simulink model "sg"  (R2021b)
settings: Solver=ode4  StartTime=0.0  StopTime=10  FixedStep=Ts  RelTol=1e-3  EnableMultiTasking=on
model workspace (MAT data in the model file):
  AU1 = 0.174532925199
  AU2 = 0
  AU3 = 0
  AW = 0
  FU1 = 0.1
  FU2 = 0
  FU3 = 0
  FW = 0
  GainU1 = 1
  GainU2 = 1
  GainU3 = 1
  GainW = 1
  KD1 = 0
  KD2 = 0
  KD3 = 0
  KI1 = 0
  KI2 = 0
  KI3 = 0
  KP1 = 1
  KP2 = 1
  KP3 = 1
  N1 = 100
  N2 = 100
  N3 = 100
  SatU1 = 0.174532920122
  SatU2 = 0.174532920122
  SatU3 = 0.174532920122
  SatW = 0.300000011921
  controlMode = 0
  qref = [0.698131680489; -0.523598790169; -1.57079637051]
libraries: slpidlib x3, slrealtimeutilitieslib x2, slrealtimeiplib x2
settings Model: Creator=ronnyl10  LastModifiedBy=Mechatronics_lab
settings SolverCC: ConcurrentTasks=on  AlgebraicLoopSolver=TrustRegion  PositivePriorityOrder=on  InsertRTBMode=Never (minimum delay)
settings DataIOCC: ExternalInput=ds  LoadExternalInput=on  SaveFormat=Array  SaveState=on  SignalLoggingName=logsOut
settings OptimizationCC: BlockReduction=off  BooleanDataType=off  OptimizeBlockIOStorage=off  BufferReuse=off  GlobalBufferReuse=off  ExpressionFolding=off  LocalBlockOutputs=off  InitFltsAndDblsToZero=on  OptimizeDataStoreBuffers=off  BusAssignmentInplaceUpdate=off
settings DebuggingCC: SaveWithParameterizedLinksMsg=none  UnderspecifiedInitializationDetection=Classic  MergeDetectMultiDrivingBlocksExec=none  CheckExecutionContextPreStartOutputMsg=on  SignalResolutionControl=TryResolveAllWithWarning  TasksWithSamePriorityMsg=none  SFUnexpectedBacktrackingDiag=warning  SFNoUnconditionalDefaultTransitionDiag=warning  SFExecutionAtInitializationDiag=none  SFMachineParentedDataDiag=warning  ArithmeticOperatorsInVariantConditions=warning
settings HardwareCC: ProdBitPerLong=64  ProdLongLongMode=on  ProdHWDeviceType=Intel->x86-64 (Linux 64)
settings ModelReferenceCC: PropagateSignalLabelsOutOfModel=off
settings SFSimCC: SimUseLocalCustomCode=off  SimTargetLang=C++
settings RTWCC: Description=Simulink Real-Time  SystemTargetFile=slrealtime.tlc  TemplateMakefile=slrealtime_default_tmf  RTWVerbose=off  RTWUseLocalCustomCode=off  Toolchain=Simulink Real-Time Toolchain  BuildConfiguration=Faster Runs  CodeExecutionProfiling=on  TargetLang=C++
settings CodeAppCC: StateflowObjectComments=on
settings SimulinkRealTimeTargetCC: MATLABClassNameForMDSCustomization=Simulink.SoftwareTarget.GRTCustomization  UseGCCFastMath=on
settings ConfigComp: CovMetricSettings=dw  CovSaveCumulativeToWorkspaceVar=on  CovSaveSingleToWorkspaceVar=on  CovExternalEMLEnable=off  CovSFcnEnable=off

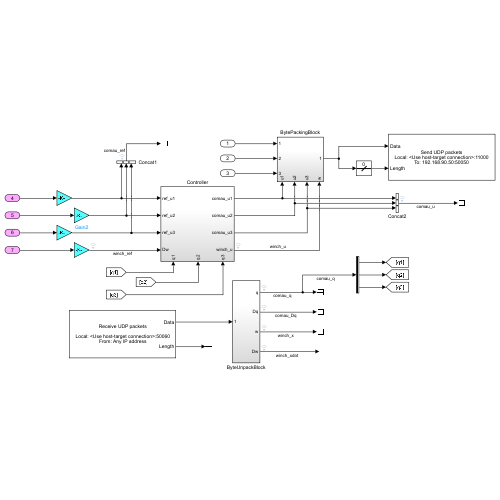
[thumbnail: Simulink's stored preview of the top-level diagram]
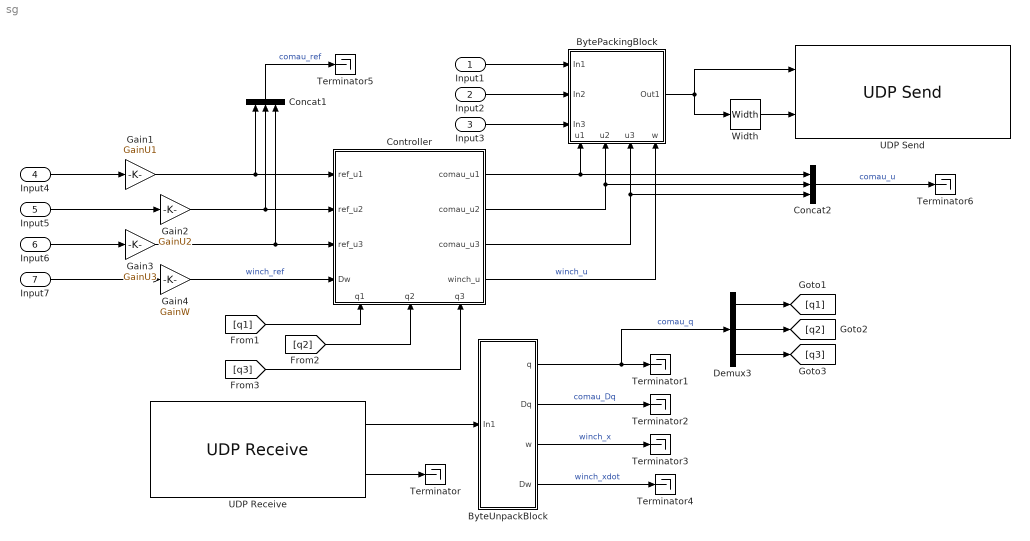
== system sg ==
  Input1 : Inport  OutDataTypeStr=uint32
  Input2 : Inport  Port=2  OutDataTypeStr=single
  Input3 : Inport  Port=3  OutDataTypeStr=single
  Input4 : Inport  Port=4  OutDataTypeStr=single  LockScale=on
  Input5 : Inport  Port=5  OutDataTypeStr=single  LockScale=on
  Input6 : Inport  Port=6  OutDataTypeStr=single  LockScale=on
  Input7 : Inport  Port=7  OutDataTypeStr=single
  BytePackingBlock : Subsystem
      settings: PortSchema="{\"entries\":[{\"content\":{\"sides\":[{\"content\":{\"connectorIds\":[\"In1\",\"In2\",\"In3\"]},\"type\":\"ConnectorPlacement.EquallySpacedRectSide\",\"uuid\":\"2ce4a3a0-ffcc-43d7-9a0a-8eda699e79f7\"},{\"content\":{\"connectorIds\":[\"Out1\"],\"side\":\"RIGHT\"},\"type\":\"ConnectorPlacement.EquallySpacedRectSide\",\"uuid\":\"6b0835cb-1c02-4104-b44f-3bd25ad1f1a4\"},{\"content\":{\"connectorIds\":[],\"side\":\"TOP\"},\"type\":\"ConnectorPlacement.EquallySpacedRectSide\",\"uuid\":\"5708f016-a603-4602-bfb0-c60eac1ca3fe\"},{\"content\":{\"connectorIds\":[\"In4\",\"In5\",\"In6\",\"In7\"],\"side\":\"BOTTOM\"},\"type\":\"ConnectorPlacement.EquallySpacedRectSide\",\"uuid\":\"ec76ed57-869b-40d0-9db7-9ec796597bae\"}]},\"type\":\"ConnectorPlacement.EquallySpacedConnector\",\"uuid\":\"dfe3046e-e9d4-4a64-bd13-28ebfaf09d3c\"}],\"packageUris\":[\"http://schema.mathworks.com/mf0/Connector/R2020b\"],\"version\":\"1.0\"}"
  ByteUnpackBlock : Subsystem
  Concat1 : Concatenate  NumInputs=3  ConcatenateDimension=2
  Concat2 : Concatenate  NumInputs=3  ConcatenateDimension=2
  Controller : Subsystem
      settings: PortSchema="{\"entries\":[{\"content\":{\"sides\":[{\"content\":{\"connectorIds\":[\"In1\",\"In2\",\"In3\",\"In4\"]},\"type\":\"ConnectorPlacement.EquallySpacedRectSide\",\"uuid\":\"8cd68c6a-417b-4593-9fd2-f26242799ae2\"},{\"content\":{\"connectorIds\":[\"Out1\",\"Out2\",\"Out3\",\"Out4\"],\"side\":\"RIGHT\"},\"type\":\"ConnectorPlacement.EquallySpacedRectSide\",\"uuid\":\"847d4d9d-1a2d-44bd-a0b5-d0f29db0c6e7\"},{\"content\":{\"connectorIds\":[],\"side\":\"TOP\"},\"type\":\"ConnectorPlacement.EquallySpacedRectSide\",\"uuid\":\"bbe996aa-4357-46c2-b640-27c97a1f9741\"},{\"content\":{\"connectorIds\":[\"In5\",\"In6\",\"In7\"],\"side\":\"BOTTOM\"},\"type\":\"ConnectorPlacement.EquallySpacedRectSide\",\"uuid\":\"3733f1bb-3723-42d5-ab99-3fe4b1c5b9a3\"}]},\"type\":\"ConnectorPlacement.EquallySpacedConnector\",\"uuid\":\"cdb9b215-90f3-4ef7-bdcb-b6cb1e13a832\"}],\"packageUris\":[\"http://schema.mathworks.com/mf0/Connector/R2020b\"],\"version\":\"1.0\"}"
  Demux3 : Demux  Outputs=3
  Gain1 : Gain  Gain=GainU1  OutDataTypeStr=single
  Gain2 : Gain  Gain=GainU2  OutDataTypeStr=single
  Gain3 : Gain  Gain=GainU3  OutDataTypeStr=single
  Gain4 : Gain  Gain=GainW  OutDataTypeStr=single
  Terminator{,1..6} (7 alike) : Terminator
  UDP Receive : slrealtimeiplib/UDP Receive  useHostTargetConn=on  ipAddress=192.168.90.60  localPort=50060  rcvWidth=304  rcvFmAny=on  fmAddress=192.168.90.50  sampleTime=Ts
      settings: SourceProductBaseCode=XP
  UDP Send : slrealtimeiplib/UDP Send  useHostTargetConn=on  toAddress=192.168.90.50  toPort=50050  sampleTime=Ts  localPort=11000
      settings: SourceProductBaseCode=XP
  Width : Width
  wires:
  Width/1 -> UDP Send/2
  UDP Receive/2 -> Terminator/1
  Concat2/1 -> Terminator6/1  "comau_u"
  BytePackingBlock/1(Out1) -> Width/1, UDP Send/1
  Input1/1 -> BytePackingBlock/1(In1)
  Input3/1 -> BytePackingBlock/3(In3)
  Input2/1 -> BytePackingBlock/2(In2)
  UDP Receive/1 -> ByteUnpackBlock/1(In1)
  Input4/1 -> Gain1/1
  Input5/1 -> Gain2/1
  Input6/1 -> Gain3/1
  ByteUnpackBlock/3(w) -> Terminator3/1  "winch_x"
  ByteUnpackBlock/4(Dw) -> Terminator4/1  "winch_xdot"
  Controller/3(comau_u3) -> Concat2/3, BytePackingBlock/6(u3)
  Controller/2(comau_u2) -> Concat2/2, BytePackingBlock/5(u2)
  Controller/1(comau_u1) -> BytePackingBlock/4(u1), Concat2/1
  Concat1/1 -> Terminator5/1  "comau_ref"
  Controller/4(winch_u) -> BytePackingBlock/7(w)  "winch_u"
  ByteUnpackBlock/2(Dq) -> Terminator2/1  "comau_Dq"
  Input7/1 -> Gain4/1
  Gain4/1 -> Controller/4(Dw)  "winch_ref"
  Gain1/1 -> Concat1/1, Controller/1(ref_u1)
  Gain2/1 -> Controller/2(ref_u2), Concat1/2
  Gain3/1 -> Concat1/3, Controller/3(ref_u3)
  ByteUnpackBlock/1(q) -> Demux3/1, Terminator1/1  "comau_q"
  Demux3/1 -> [q1]
  Demux3/2 -> [q2]
  Demux3/3 -> [q3]
  [q2] -> Controller/6(q2)
  [q3] -> Controller/7(q3)
  [q1] -> Controller/5(q1)

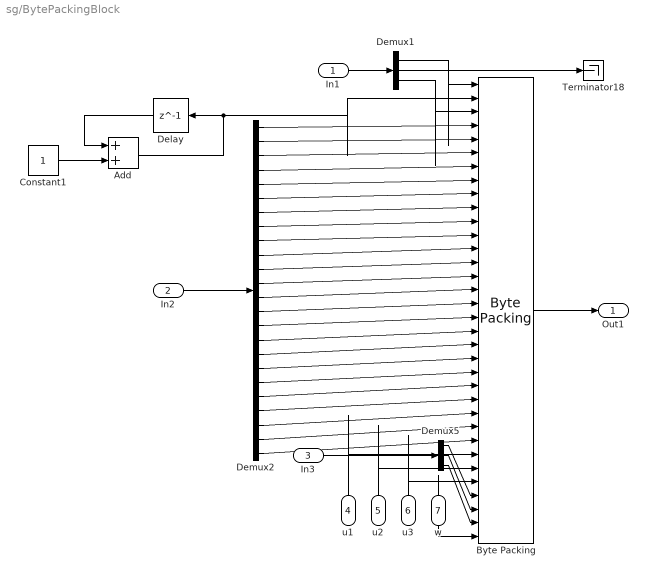
== system sg/BytePackingBlock ==
  In1 : Inport
  In2 : Inport  Port=2
  In3 : Inport  Port=3
  u1 : Inport  Port=4
  u2 : Inport  Port=5
  u3 : Inport  Port=6
  w : Inport  Port=7
  Add : Sum
  Byte Packing : slrealtimeutilitieslib/Byte Packing  MaskPackedDataType=uint8  MaskUnpackedDataTypes={'uint32', 'uint32', 'uint32', 'single', 'single', 'single', 'single', 'single', 'single', 'single', 'single', 'single', 'single', 'single', 'single', 'single', 'single', 'single', 'single', 'single', 'single', 'single', 'single', 'single', 'single', 'single', 'single', 'single', 'single', 'single', 'single', 'single', 'single', 'single'}  MaskAlignment=1
  Constant1 : Constant  OutDataTypeStr=uint32
  Delay : Delay  DelayLength=1
  Demux1 : Demux  Outputs=3
  Demux2 : Demux  Outputs=24
  Demux5 : Demux  Outputs=3
  Terminator18 : Terminator
  Out1 : Outport
  wires:
  Demux2/19 -> Byte Packing/22
  Demux2/21 -> Byte Packing/24
  u3/1 -> Byte Packing/30
  Demux2/2 -> Byte Packing/5
  u2/1 -> Byte Packing/29
  Demux5/1 -> Byte Packing/31
  Demux5/2 -> Byte Packing/32
  Demux1/3 -> Byte Packing/3
  In2/1 -> Demux2/1
  Demux2/22 -> Byte Packing/25
  Demux2/1 -> Byte Packing/4
  Demux2/15 -> Byte Packing/18
  Demux2/18 -> Byte Packing/21
  Delay/1 -> Add/1
  Demux2/24 -> Byte Packing/27
  Demux1/2 -> Terminator18/1
  In1/1 -> Demux1/1
  Demux2/5 -> Byte Packing/8
  Add/1 -> Byte Packing/2, Delay/1
  Constant1/1 -> Add/2
  Demux2/6 -> Byte Packing/9
  Demux2/9 -> Byte Packing/12
  Demux2/10 -> Byte Packing/13
  Demux2/20 -> Byte Packing/23
  Demux2/8 -> Byte Packing/11
  Demux2/12 -> Byte Packing/15
  Demux2/23 -> Byte Packing/26
  Demux2/16 -> Byte Packing/19
  Demux1/1 -> Byte Packing/1
  Demux5/3 -> Byte Packing/33
  Demux2/3 -> Byte Packing/6
  Demux2/11 -> Byte Packing/14
  Demux2/7 -> Byte Packing/10
  Demux2/4 -> Byte Packing/7
  Demux2/13 -> Byte Packing/16
  Demux2/17 -> Byte Packing/20
  Demux2/14 -> Byte Packing/17
  u1/1 -> Byte Packing/28
  In3/1 -> Demux5/1
  Byte Packing/1 -> Out1/1
  w/1 -> Byte Packing/34

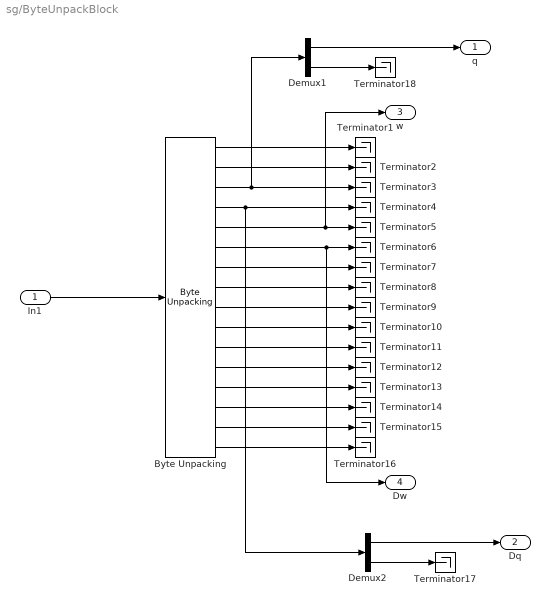
== system sg/ByteUnpackBlock ==
  In1 : Inport
  Byte Unpacking : slrealtimeutilitieslib/Byte Unpacking  MaskUnpackedDataTypes={'uint32', 'single', 'single', 'single', 'single', 'single', 'single', 'single', 'single', 'single', 'single', 'single', 'single', 'single', 'single', 'single'}  MaskUnpackedDataSizes={[1], [1], [6], [6], [1], [1], [6], [6], [6], [6], [6], [6], [6], [6], [6], [6]}  MaskAlignment=1
      settings: SourceProductBaseCode=XP
  Demux1 : Demux  Outputs=2
  Demux2 : Demux  Outputs=2
  Terminator{1..18} (18 alike) : Terminator
  q : Outport
  Dq : Outport  Port=2
  w : Outport  Port=3
  Dw : Outport  Port=4
  wires:
  Byte Unpacking/13 -> Terminator13/1
  Byte Unpacking/8 -> Terminator8/1
  Byte Unpacking/1 -> Terminator1/1
  Byte Unpacking/7 -> Terminator7/1
  Byte Unpacking/16 -> Terminator16/1
  Byte Unpacking/6 -> Terminator6/1, Dw/1
  Byte Unpacking/11 -> Terminator11/1
  Byte Unpacking/10 -> Terminator10/1
  Byte Unpacking/15 -> Terminator15/1
  Byte Unpacking/2 -> Terminator2/1
  Byte Unpacking/14 -> Terminator14/1
  Byte Unpacking/5 -> w/1, Terminator5/1
  Byte Unpacking/9 -> Terminator9/1
  Byte Unpacking/12 -> Terminator12/1
  In1/1 -> Byte Unpacking/1
  Demux1/1 -> q/1
  Byte Unpacking/3 -> Demux1/1, Terminator3/1
  Demux2/1 -> Dq/1
  Byte Unpacking/4 -> Demux2/1, Terminator4/1
  Demux1/2 -> Terminator18/1
  Demux2/2 -> Terminator17/1

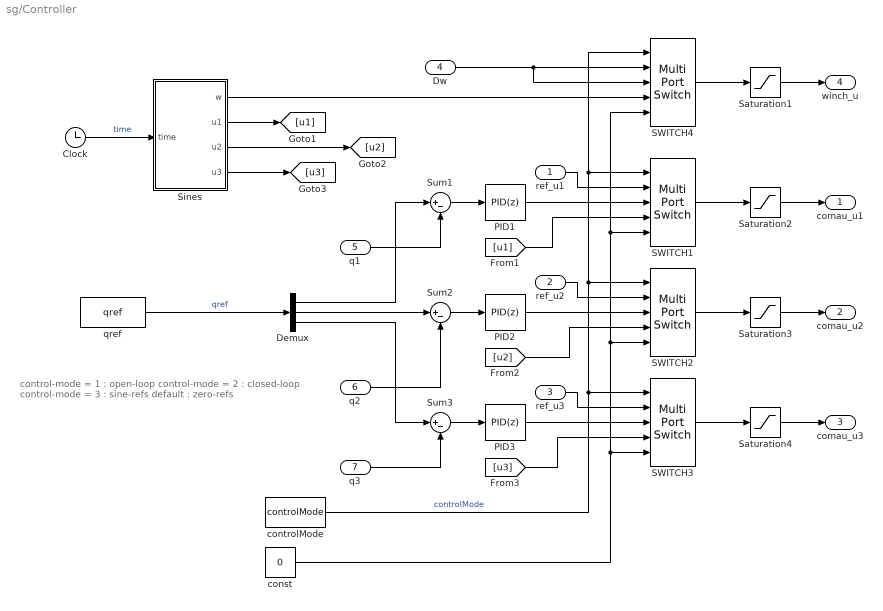
== system sg/Controller ==
  note: control-mode = 1 : open-loop
      | control-mode = 2 : closed-loop
      | control-mode = 3 : sine-refs
      | default : zero-refs
  ref_u1 : Inport
  ref_u2 : Inport  Port=2
  ref_u3 : Inport  Port=3
  Dw : Inport  Port=4
  q1 : Inport  Port=5
  q2 : Inport  Port=6
  q3 : Inport  Port=7
  Clock : Clock
  Demux : Demux  Outputs=3
  PID1 : slpidlib/PID Controller  Controller=PID  Form=Parallel  TimeDomain=Discrete-time  UseExternalTs=off  SampleTime=-1  IntegratorMethod=Forward Euler  FilterMethod=Forward Euler  ControllerParametersSource=internal  P=KP1  I=KI1  D=KD1  UseFilter=on  N=N1  TunerSelectOption=Transfer Function Based (PID Tuner App)  InitialConditionSource=internal  InitialConditionForIntegrator=0  InitialConditionForFilter=0  DifferentiatorICPrevScaledInput=0  ExternalReset=none  TrackingMode=off  Kt=1  LimitOutput=off  SatLimitsSource=internal  UpperSaturationLimit=inf  LowerSaturationLimit=-inf  LinearizeAsGain=on  AntiWindupMode=none  Kb=1  POutMin=[]  POutMax=[]  IOutMin=[]  IOutMax=[]  DOutMin=[]  DOutMax=[]  NOutMin=[]  NOutMax=[]  SumOutMin=[]  SumOutMax=[]  SaturationOutMin=[]  SaturationOutMax=[]  PParamMin=[]  PParamMax=[]  IParamMin=[]  IParamMax=[]  DParamMin=[]  DParamMax=[]  NParamMin=[]  NParamMax=[]  KbParamMin=[]  KbParamMax=[]  KtParamMin=[]  KtParamMax=[]  KbOutMin=[]  KbOutMax=[]  KtOutMin=[]  KtOutMax=[]  IntegratorOutMin=[]  IntegratorOutMax=[]  FilterOutMin=[]  FilterOutMax=[]  SumI1OutMin=[]  SumI1OutMax=[]  SumI2OutMin=[]  SumI2OutMax=[]  SumI3OutMin=[]  SumI3OutMax=[]  SumI4OutMin=[]  SumI4OutMax=[]  SumDOutMin=[]  SumDOutMax=[]  DifferentiatorOutMin=[]  DifferentiatorOutMax=[]  FilterDiffOutCoefMin=[]  FilterDiffOutCoefMax=[]  ReciprocalOutMin=[]  ReciprocalOutMax=[]  SumDenOutMin=[]  SumDenOutMax=[]  SumNumOutMin=[]  SumNumOutMax=[]  DivideOutMin=[]  DivideOutMax=[]  UdiffTsProdOutMin=[]  UdiffTsProdOutMax=[]  NTsProdOutMin=[]  NTsProdOutMax=[]  UintegralTsProdOutMin=[]  UintegralTsProdOutMax=[]  UngainTsProdOutMin=[]  UngainTsProdOutMax=[]  FilterDenConstantOutDataTypeStr=Inherit: Inherit via back propagation  FilterDenConstantOutMin=[]  FilterDenConstantOutMax=[]  PCopyOutDataTypeStr=Inherit: Inherit via back propagation  PCopyOutMin=[]  PCopyOutMax=[]  NCopyOutDataTypeStr=Inherit: Inherit via back propagation  NCopyOutMin=[]  NCopyOutMax=[]  IntegratorContinuousStateAttributes=''  IntegratorStateMustResolveToSignalObject=off  IntegratorRTWStateStorageClass=Auto  FilterContinuousStateAttributes=''  FilterStateMustResolveToSignalObject=off  FilterRTWStateStorageClass=Auto  ParallelPVariant=InternalParameters  IdealPVariant=Disabled  IVariant=InternalParameters  DVariant=InternalParameters  IntegratorVariant=Discrete  SatVariant=Disabled  AWVariant=Passthrough  PCopyVariant=Disabled  TRVariant=Disabled  FdbkBlocksVariant=Forward  IdealPFdbkVariant=Disabled  SatFdbkVariant=Disabled  DerivativeFilterVariant=ForwardEulerFilter  NVariant=InternalParameters  NCopyVariant=Disabled  FilterICVariant=InternalICsFilter  IntegratorICVariant=InternalICs  ExternalResetVariant=Disabled  TRSumVariant=Passthrough  SumFdbkVariant=Disabled  SumVariant=Sum_PID  TsampFilterVariant=InternalTs  TsampNgainVariant=Passthrough  TsampIntegralVariant=Passthrough  ExternalSaturationOutDataTypeStr=Inherit: Same as second input
  PID2 : slpidlib/PID Controller  Controller=PID  Form=Parallel  TimeDomain=Discrete-time  UseExternalTs=off  SampleTime=-1  IntegratorMethod=Forward Euler  FilterMethod=Forward Euler  ControllerParametersSource=internal  P=KP2  I=KI2  D=KD2  UseFilter=on  N=N2  TunerSelectOption=Transfer Function Based (PID Tuner App)  InitialConditionSource=internal  InitialConditionForIntegrator=0  InitialConditionForFilter=0  DifferentiatorICPrevScaledInput=0  ExternalReset=none  TrackingMode=off  Kt=1  LimitOutput=off  SatLimitsSource=internal  UpperSaturationLimit=inf  LowerSaturationLimit=-inf  LinearizeAsGain=on  AntiWindupMode=none  Kb=1  POutMin=[]  POutMax=[]  IOutMin=[]  IOutMax=[]  DOutMin=[]  DOutMax=[]  NOutMin=[]  NOutMax=[]  SumOutMin=[]  SumOutMax=[]  SaturationOutMin=[]  SaturationOutMax=[]  PParamMin=[]  PParamMax=[]  IParamMin=[]  IParamMax=[]  DParamMin=[]  DParamMax=[]  NParamMin=[]  NParamMax=[]  KbParamMin=[]  KbParamMax=[]  KtParamMin=[]  KtParamMax=[]  KbOutMin=[]  KbOutMax=[]  KtOutMin=[]  KtOutMax=[]  IntegratorOutMin=[]  IntegratorOutMax=[]  FilterOutMin=[]  FilterOutMax=[]  SumI1OutMin=[]  SumI1OutMax=[]  SumI2OutMin=[]  SumI2OutMax=[]  SumI3OutMin=[]  SumI3OutMax=[]  SumI4OutMin=[]  SumI4OutMax=[]  SumDOutMin=[]  SumDOutMax=[]  DifferentiatorOutMin=[]  DifferentiatorOutMax=[]  FilterDiffOutCoefMin=[]  FilterDiffOutCoefMax=[]  ReciprocalOutMin=[]  ReciprocalOutMax=[]  SumDenOutMin=[]  SumDenOutMax=[]  SumNumOutMin=[]  SumNumOutMax=[]  DivideOutMin=[]  DivideOutMax=[]  UdiffTsProdOutMin=[]  UdiffTsProdOutMax=[]  NTsProdOutMin=[]  NTsProdOutMax=[]  UintegralTsProdOutMin=[]  UintegralTsProdOutMax=[]  UngainTsProdOutMin=[]  UngainTsProdOutMax=[]  FilterDenConstantOutDataTypeStr=Inherit: Inherit via back propagation  FilterDenConstantOutMin=[]  FilterDenConstantOutMax=[]  PCopyOutDataTypeStr=Inherit: Inherit via back propagation  PCopyOutMin=[]  PCopyOutMax=[]  NCopyOutDataTypeStr=Inherit: Inherit via back propagation  NCopyOutMin=[]  NCopyOutMax=[]  IntegratorContinuousStateAttributes=''  IntegratorStateMustResolveToSignalObject=off  IntegratorRTWStateStorageClass=Auto  FilterContinuousStateAttributes=''  FilterStateMustResolveToSignalObject=off  FilterRTWStateStorageClass=Auto  ParallelPVariant=InternalParameters  IdealPVariant=Disabled  IVariant=InternalParameters  DVariant=InternalParameters  IntegratorVariant=Discrete  SatVariant=Disabled  AWVariant=Passthrough  PCopyVariant=Disabled  TRVariant=Disabled  FdbkBlocksVariant=Forward  IdealPFdbkVariant=Disabled  SatFdbkVariant=Disabled  DerivativeFilterVariant=ForwardEulerFilter  NVariant=InternalParameters  NCopyVariant=Disabled  FilterICVariant=InternalICsFilter  IntegratorICVariant=InternalICs  ExternalResetVariant=Disabled  TRSumVariant=Passthrough  SumFdbkVariant=Disabled  SumVariant=Sum_PID  TsampFilterVariant=InternalTs  TsampNgainVariant=Passthrough  TsampIntegralVariant=Passthrough  ExternalSaturationOutDataTypeStr=Inherit: Same as second input
  PID3 : slpidlib/PID Controller  Controller=PID  Form=Parallel  TimeDomain=Discrete-time  UseExternalTs=off  SampleTime=-1  IntegratorMethod=Forward Euler  FilterMethod=Forward Euler  ControllerParametersSource=internal  P=KP3  I=KI3  D=KD3  UseFilter=on  N=N3  TunerSelectOption=Transfer Function Based (PID Tuner App)  InitialConditionSource=internal  InitialConditionForIntegrator=0  InitialConditionForFilter=0  DifferentiatorICPrevScaledInput=0  ExternalReset=none  TrackingMode=off  Kt=1  LimitOutput=off  SatLimitsSource=internal  UpperSaturationLimit=inf  LowerSaturationLimit=-inf  LinearizeAsGain=on  AntiWindupMode=none  Kb=1  POutMin=[]  POutMax=[]  IOutMin=[]  IOutMax=[]  DOutMin=[]  DOutMax=[]  NOutMin=[]  NOutMax=[]  SumOutMin=[]  SumOutMax=[]  SaturationOutMin=[]  SaturationOutMax=[]  PParamMin=[]  PParamMax=[]  IParamMin=[]  IParamMax=[]  DParamMin=[]  DParamMax=[]  NParamMin=[]  NParamMax=[]  KbParamMin=[]  KbParamMax=[]  KtParamMin=[]  KtParamMax=[]  KbOutMin=[]  KbOutMax=[]  KtOutMin=[]  KtOutMax=[]  IntegratorOutMin=[]  IntegratorOutMax=[]  FilterOutMin=[]  FilterOutMax=[]  SumI1OutMin=[]  SumI1OutMax=[]  SumI2OutMin=[]  SumI2OutMax=[]  SumI3OutMin=[]  SumI3OutMax=[]  SumI4OutMin=[]  SumI4OutMax=[]  SumDOutMin=[]  SumDOutMax=[]  DifferentiatorOutMin=[]  DifferentiatorOutMax=[]  FilterDiffOutCoefMin=[]  FilterDiffOutCoefMax=[]  ReciprocalOutMin=[]  ReciprocalOutMax=[]  SumDenOutMin=[]  SumDenOutMax=[]  SumNumOutMin=[]  SumNumOutMax=[]  DivideOutMin=[]  DivideOutMax=[]  UdiffTsProdOutMin=[]  UdiffTsProdOutMax=[]  NTsProdOutMin=[]  NTsProdOutMax=[]  UintegralTsProdOutMin=[]  UintegralTsProdOutMax=[]  UngainTsProdOutMin=[]  UngainTsProdOutMax=[]  FilterDenConstantOutDataTypeStr=Inherit: Inherit via back propagation  FilterDenConstantOutMin=[]  FilterDenConstantOutMax=[]  PCopyOutDataTypeStr=Inherit: Inherit via back propagation  PCopyOutMin=[]  PCopyOutMax=[]  NCopyOutDataTypeStr=Inherit: Inherit via back propagation  NCopyOutMin=[]  NCopyOutMax=[]  IntegratorContinuousStateAttributes=''  IntegratorStateMustResolveToSignalObject=off  IntegratorRTWStateStorageClass=Auto  FilterContinuousStateAttributes=''  FilterStateMustResolveToSignalObject=off  FilterRTWStateStorageClass=Auto  ParallelPVariant=InternalParameters  IdealPVariant=Disabled  IVariant=InternalParameters  DVariant=InternalParameters  IntegratorVariant=Discrete  SatVariant=Disabled  AWVariant=Passthrough  PCopyVariant=Disabled  TRVariant=Disabled  FdbkBlocksVariant=Forward  IdealPFdbkVariant=Disabled  SatFdbkVariant=Disabled  DerivativeFilterVariant=ForwardEulerFilter  NVariant=InternalParameters  NCopyVariant=Disabled  FilterICVariant=InternalICsFilter  IntegratorICVariant=InternalICs  ExternalResetVariant=Disabled  TRSumVariant=Passthrough  SumFdbkVariant=Disabled  SumVariant=Sum_PID  TsampFilterVariant=InternalTs  TsampNgainVariant=Passthrough  TsampIntegralVariant=Passthrough  ExternalSaturationOutDataTypeStr=Inherit: Same as second input
  SWITCH1 : MultiPortSwitch  DataPortForDefault=Additional data port
  SWITCH2 : MultiPortSwitch  DataPortForDefault=Additional data port
  SWITCH3 : MultiPortSwitch  DataPortForDefault=Additional data port
  SWITCH4 : MultiPortSwitch  DataPortIndices={1,3}  DataPortForDefault=Additional data port
  Saturation1 : Saturate  UpperLimit=SatW  LowerLimit=-SatW
  Saturation2 : Saturate  UpperLimit=SatU1  LowerLimit=-SatU1
  Saturation3 : Saturate  UpperLimit=SatU2  LowerLimit=-SatU2
  Saturation4 : Saturate  UpperLimit=SatU3  LowerLimit=-SatU3
  Sines : Subsystem
  Sum1 : Sum  Inputs=|+-
  Sum2 : Sum  Inputs=|+-
  Sum3 : Sum  Inputs=|+-
  const : Constant  Value=0  OutDataTypeStr=single
  controlMode : Constant  Value=controlMode  OutDataTypeStr=double
  qref : Constant  Value=qref
  comau_u1 : Outport
  comau_u2 : Outport  Port=2
  comau_u3 : Outport  Port=3
  winch_u : Outport  Port=4
  wires:
  Saturation1/1 -> winch_u/1
  Saturation2/1 -> comau_u1/1
  Saturation3/1 -> comau_u2/1
  Saturation4/1 -> comau_u3/1
  q2/1 -> Sum2/2
  q3/1 -> Sum3/2
  Demux/1 -> Sum1/1
  q1/1 -> Sum1/2
  Sum1/1 -> PID1/1
  Sum2/1 -> PID2/1
  PID3/1 -> SWITCH3/3
  Demux/3 -> Sum3/1
  Sum3/1 -> PID3/1
  [u3] -> SWITCH3/4
  PID2/1 -> SWITCH2/3
  [u2] -> SWITCH2/4
  PID1/1 -> SWITCH1/3
  [u1] -> SWITCH1/4
  const/1 -> SWITCH4/5, SWITCH1/5, SWITCH2/5, SWITCH3/5
  SWITCH4/1 -> Saturation1/1
  SWITCH1/1 -> Saturation2/1
  SWITCH2/1 -> Saturation3/1
  SWITCH3/1 -> Saturation4/1
  Dw/1 -> SWITCH4/3, SWITCH4/2
  controlMode/1 -> SWITCH3/1, SWITCH2/1, SWITCH4/1, SWITCH1/1  "controlMode"
  ref_u1/1 -> SWITCH1/2
  qref/1 -> Demux/1  "qref"
  ref_u2/1 -> SWITCH2/2
  ref_u3/1 -> SWITCH3/2
  Demux/2 -> Sum2/1
  Clock/1 -> Sines/1(time)  "time"
  Sines/2(u1) -> [u1]
  Sines/1(w) -> SWITCH4/4
  Sines/3(u2) -> [u2]
  Sines/4(u3) -> [u3]

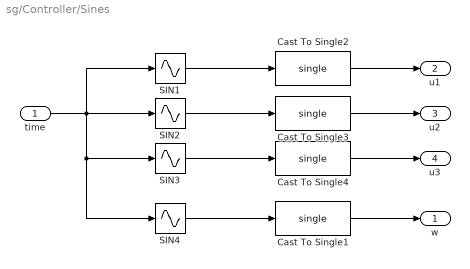
== system sg/Controller/Sines ==
  time : Inport
  Cast To Single{1..4} (4 alike) : DataTypeConversion  OutDataTypeStr=single
  SIN1 : Sin  TimeSource=Use external signal  Amplitude=AU1  Frequency=FU1*2*pi  SampleTime=0
  SIN2 : Sin  TimeSource=Use external signal  Amplitude=AU2  Frequency=FU2*2*pi  SampleTime=0
  SIN3 : Sin  TimeSource=Use external signal  Amplitude=AU3  Frequency=FU3*2*pi  SampleTime=0
  SIN4 : Sin  TimeSource=Use external signal  Amplitude=AW  Frequency=FW*2*pi  SampleTime=0
  w : Outport
  u1 : Outport  Port=2
  u2 : Outport  Port=3
  u3 : Outport  Port=4
  wires:
  Cast To Single3/1 -> u2/1
  SIN1/1 -> Cast To Single2/1
  time/1 -> SIN4/1, SIN3/1, SIN1/1, SIN2/1
  SIN4/1 -> Cast To Single1/1
  SIN2/1 -> Cast To Single3/1
  SIN3/1 -> Cast To Single4/1
  Cast To Single4/1 -> u3/1
  Cast To Single1/1 -> w/1
  Cast To Single2/1 -> u1/1
